simulink model "pwr_measure_testbench"  (R2012b)
settings: Solver=ode45  StartTime=0.0  StopTime=100000  RelTol=1e-3
undefined symbols (not defined in the file): ln
libraries: xbsIndex_r4 x64, simulink x1
settings Model: Creator=rng  LastModifiedBy=rng

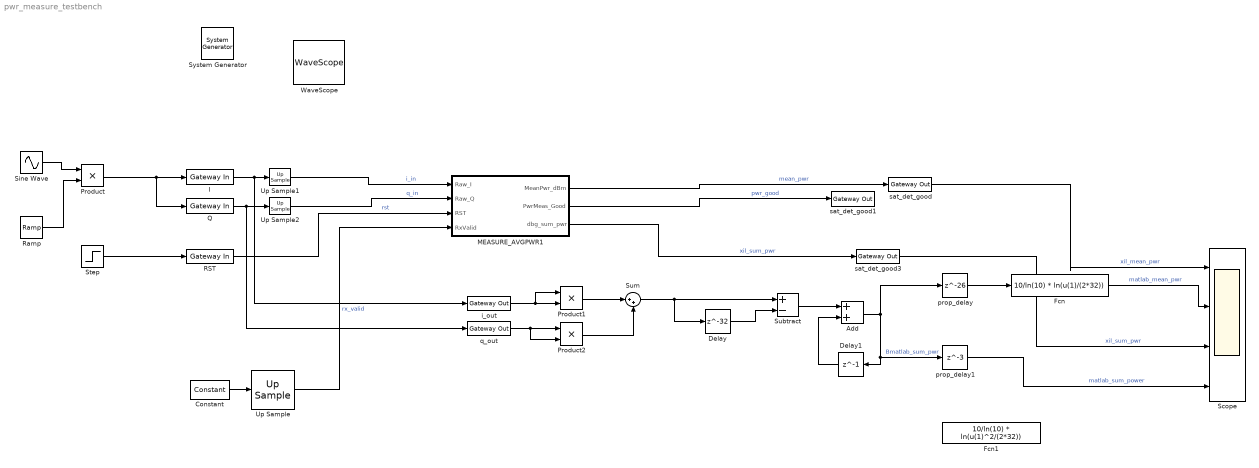
== system pwr_measure_testbench ==
  " System Generator" : xbsIndex_r4/ System Generator  Tag=genX  xilinxfamily=virtex6  part=xc6vlx240t  speed=-2  package=ff1156  synthesis_tool=XST  clock_wrapper=Clock Enables  directory=./volo_agcdc_generated_pcores  proj_type=Project Navigator  Synth_file=XST Defaults  Impl_file=ISE Defaults  testbench=off  simulink_period=1  sysclk_period=10  dcm_input_clock_period=100  incr_netlist=off  trim_vbits=Everywhere in SubSystem  dbl_ovrd=According to Block Masks  core_generation=According to Block Masks  run_coregen=off  deprecated_control=off  eval_field=0  block_type=sysgen
      settings: block_version=10.1.3
  Add : Sum
  Constant : xbsIndex_r4/Constant  const=1  gui_display_data_type=Boolean  arith_type=Boolean  n_bits=16  bin_pt=14  preci_type=Single  exp_width=8  frac_width=24  explicit_period=on  period=4  equ=P=C  opselect=C  inp2=PCIN>>17  opr=+  inp1=P  carry=CIN  dbl_ovrd=off  block_type=constant
  Delay : Delay  DelayLength=32  InitialCondition=0
  Delay1 : Delay  DelayLength=1  InitialCondition=0
  Fcn : Fcn  Expr=10/ln(10) * ln(u(1)/(2*32))
  Fcn1 : Fcn  Expr=10/ln(10) * ln(u(1)^2/(2*32))
  I : xbsIndex_r4/Gateway In  gui_display_data_type=Fixed-point  arith_type="Signed  (2's comp)"  n_bits=12  bin_pt=11  preci_type=Single  exp_width=8  frac_width=24  quantization="Round  (unbiased: +/- Inf)"  overflow=Saturate  period=4  dbl_ovrd=off  timing_constraint=None  locs_specified=off  LOCs={}  UseAsADC=off  ADCChannel='1'  inherit_from_input=off  hdl_port=on  block_type=gatewayin
  MEASURE_AVGPWR1 : Subsystem
  Product : Product  RndMeth=Zero
  Product1 : Product  RndMeth=Zero
  Product2 : Product  RndMeth=Zero
  Q : xbsIndex_r4/Gateway In  gui_display_data_type=Fixed-point  arith_type="Signed  (2's comp)"  n_bits=12  bin_pt=11  preci_type=Single  exp_width=8  frac_width=24  quantization="Round  (unbiased: +/- Inf)"  overflow=Saturate  period=4  dbl_ovrd=off  timing_constraint=None  locs_specified=off  LOCs={}  UseAsADC=off  ADCChannel='1'  inherit_from_input=off  hdl_port=on  block_type=gatewayin
  RST : xbsIndex_r4/Gateway In  gui_display_data_type=Boolean  arith_type=Boolean  n_bits=12  bin_pt=11  preci_type=Single  exp_width=8  frac_width=24  quantization="Round  (unbiased: +/- Inf)"  overflow=Saturate  period=1  dbl_ovrd=off  timing_constraint=None  locs_specified=off  LOCs={}  UseAsADC=off  ADCChannel='1'  inherit_from_input=off  hdl_port=on  block_type=gatewayin
  Ramp : simulink/Sources/Ramp  slope=0.1  start=0  X0=0
  Scope : Scope  NumInputPorts=4
      settings: YMin=0~-5~-5~-5  YMax=0.003~5~5~5
  Sine Wave : Sin  Amplitude=0.000001  Frequency=10  SampleTime=1
  Step : Step  Time=5  Before=1  After=0  SampleTime=0
  Subtract : Sum  Inputs=+-
  Sum : Sum  Inputs=|++
  Up Sample : xbsIndex_r4/Up Sample  sample_ratio=4  copy_samples=off  en=off  latency=0  dbl_ovrd=off  block_type=usamp
  Up Sample1 : xbsIndex_r4/Up Sample  sample_ratio=4  copy_samples=on  en=off  latency=0  dbl_ovrd=off  block_type=usamp
  Up Sample2 : xbsIndex_r4/Up Sample  sample_ratio=4  copy_samples=on  en=off  latency=0  dbl_ovrd=off  block_type=usamp
  WaveScope : xbsIndex_r4/WaveScope  block_type=wavescope
  i_out : xbsIndex_r4/Gateway Out  inherit_from_input=off  hdl_port=off  timing_constraint=None  locs_specified=off  LOCs={}  UseAsDAC=off  DACChannel='1'  block_type=gatewayout
  prop_delay : Delay  DelayLength=26  InitialCondition=0
  prop_delay1 : Delay  DelayLength=3  InitialCondition=0
  q_out : xbsIndex_r4/Gateway Out  inherit_from_input=off  hdl_port=off  timing_constraint=None  locs_specified=off  LOCs={}  UseAsDAC=off  DACChannel='1'  block_type=gatewayout
  sat_det_good : xbsIndex_r4/Gateway Out  inherit_from_input=off  hdl_port=off  timing_constraint=None  locs_specified=off  LOCs={}  UseAsDAC=off  DACChannel='1'  block_type=gatewayout
  sat_det_good1 : xbsIndex_r4/Gateway Out  inherit_from_input=off  hdl_port=off  timing_constraint=None  locs_specified=off  LOCs={}  UseAsDAC=off  DACChannel='1'  block_type=gatewayout
  sat_det_good3 : xbsIndex_r4/Gateway Out  inherit_from_input=off  hdl_port=off  timing_constraint=None  locs_specified=off  LOCs={}  UseAsDAC=off  DACChannel='1'  block_type=gatewayout
  wires:
  I/1 -> i_out/1, Up Sample1/1
  Q/1 -> q_out/1, Up Sample2/1
  Constant/1 -> Up Sample/1
  Up Sample/1 -> MEASURE_AVGPWR1/4(RxValid)  "rx_valid"
  Up Sample1/1 -> MEASURE_AVGPWR1/1(Raw_I)  "i_in"
  Up Sample2/1 -> MEASURE_AVGPWR1/2(Raw_Q)  "q_in"
  Product/1 -> Q/1, I/1
  Sine Wave/1 -> Product/1
  Ramp/1 -> Product/2
  Step/1 -> RST/1
  MEASURE_AVGPWR1/1(MeanPwr_dBm) -> sat_det_good/1  "mean_pwr"
  MEASURE_AVGPWR1/2(PwrMeas_Good) -> sat_det_good1/1  "pwr_good"
  RST/1 -> MEASURE_AVGPWR1/3(RST)  "rst"
  i_out/1 -> Product1/2, Product1/1
  q_out/1 -> Product2/2, Product2/1
  Product1/1 -> Sum/1
  Product2/1 -> Sum/2
  Delay/1 -> Subtract/2
  Sum/1 -> Subtract/1, Delay/1
  Subtract/1 -> Add/1
  Add/1 -> Delay1/1, prop_delay1/1, prop_delay/1  "Bmatlab_sum_pwr"
  Delay1/1 -> Add/2
  Fcn/1 -> Scope/2  "matlab_mean_pwr"
  sat_det_good/1 -> Scope/1  "xil_mean_pwr"
  MEASURE_AVGPWR1/3(dbg_sum_pwr) -> sat_det_good3/1  "xil_sum_pwr"
  prop_delay/1 -> Fcn/1
  prop_delay1/1 -> Scope/4  "matlab_sum_power"
  sat_det_good3/1 -> Scope/3  "xil_sum_pwr"

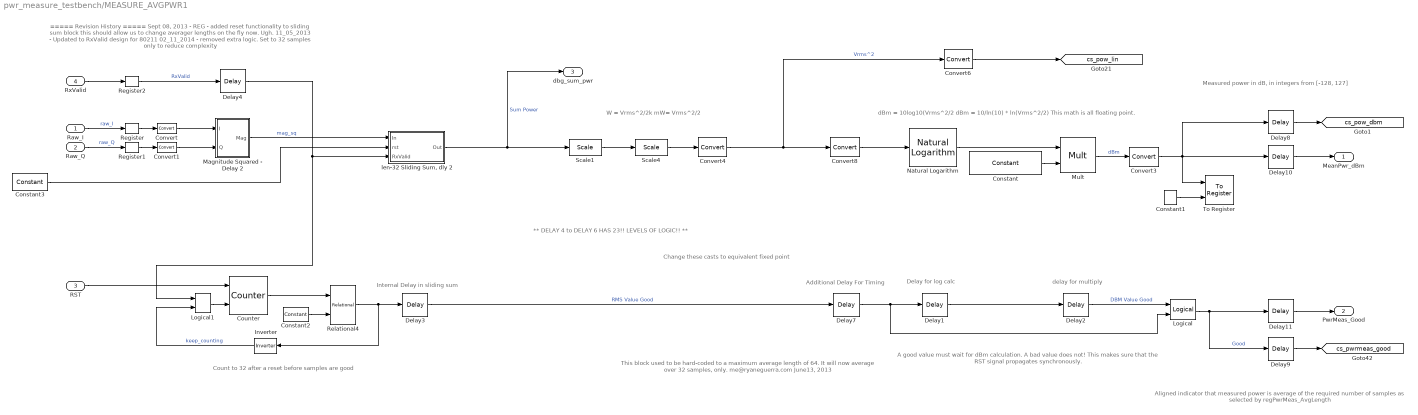
== system pwr_measure_testbench/MEASURE_AVGPWR1 ==
  note: delay for multiply
  note: Delay for log calc
  note: Count to 32 after a reset before samples are good
  note: Change these casts to equivalent fixed point
  note: ** DELAY 4 to DELAY 6 HAS 23!! LEVELS OF LOGIC!! **
  note: Additional Delay For Timing
  note: Internal Delay in sliding sum
  note: ===== Revision History =====
      | Sept 08, 2013 - REG - added reset functionality to sliding sum block
      | this should allow us to change averager lengths on the fly now. Ugh.
      | 11_05_2013 - Updated to RxValid design for 80211
      | 02_11_2014 - removed extra logic. Set to 32 samples only to reduce complexity
  note: A good value must wait for dBm calculation.
      | A bad value does not! This makes sure that
      | the RST signal propagates synchronously.
  note: Aligned indicator that
      | measured power is average
      | of the required number
      | of samples as selected
      | by regPwrMeas_AvgLength
  note: Measured power in dB,
      | in  integers from
      | [-128, 127]
  note: dBm = 10log10(Vrms^2/2
      | dBm = 10/ln(10) * ln(Vrms^2/2)
      | This math is all floating point.
  note: W = Vrms^2/2k
      | mW= Vrms^2/2
  note: This block used to be hard-coded to a maximum average length of 64.
      | It will now average over 32 samples, only.
      | me@ryaneguerra.com
      | June13, 2013
  Raw_I : Inport
  Raw_Q : Inport  Port=2
  RST : Inport  Port=3
  RxValid : Inport  Port=4
  Constant : xbsIndex_r4/Constant  const=10/log(10)  gui_display_data_type=Floating-point  arith_type=Floating-point  n_bits=18  bin_pt=14  preci_type=Single  exp_width=8  frac_width=24  explicit_period=on  period=1  equ=P=C  opselect=C  inp2=PCIN>>17  opr=+  inp1=P  carry=CIN  dbl_ovrd=off  block_type=constant
  Constant1 : xbsIndex_r4/Constant  const=1  gui_display_data_type=Boolean  arith_type=Boolean  n_bits=18  bin_pt=14  preci_type=Single  exp_width=8  frac_width=24  explicit_period=on  period=1  equ=P=C  opselect=C  inp2=PCIN>>17  opr=+  inp1=P  carry=CIN  dbl_ovrd=off  block_type=constant
  Constant2 : xbsIndex_r4/Constant  const=32  gui_display_data_type=Fixed-point  arith_type=Unsigned  n_bits=6  bin_pt=0  preci_type=Single  exp_width=8  frac_width=24  explicit_period=on  period=1  equ=P=C  opselect=C  inp2=PCIN>>17  opr=+  inp1=P  carry=CIN  dbl_ovrd=off  block_type=constant
  Constant3 : xbsIndex_r4/Constant  const=0  gui_display_data_type=Boolean  arith_type=Boolean  n_bits=16  bin_pt=14  preci_type=Single  exp_width=8  frac_width=24  explicit_period=on  period=1  equ=P=C  opselect=C  inp2=PCIN>>17  opr=+  inp1=P  carry=CIN  dbl_ovrd=off  block_type=constant
  Convert : xbsIndex_r4/Convert  gui_display_data_type=Fixed-point  arith_type="Signed  (2's comp)"  n_bits=12  bin_pt=11  float_type=Single  exp_bits=8  fraction_bits=24  quantization=Truncate  overflow=Wrap  en=off  latency=0  dbl_ovrd=off  pipeline=off  block_type=convert
  Convert1 : xbsIndex_r4/Convert  gui_display_data_type=Fixed-point  arith_type="Signed  (2's comp)"  n_bits=12  bin_pt=11  float_type=Single  exp_bits=8  fraction_bits=24  quantization=Truncate  overflow=Wrap  en=off  latency=0  dbl_ovrd=off  pipeline=off  block_type=convert
  Convert3 : xbsIndex_r4/Convert  gui_display_data_type=Fixed-point  arith_type="Signed  (2's comp)"  n_bits=9  bin_pt=0  float_type=Single  exp_bits=8  fraction_bits=24  quantization="Round  (unbiased: +/- Inf)"  overflow=Saturate  en=off  latency=0  dbl_ovrd=off  pipeline=off  block_type=convert
  Convert4 : xbsIndex_r4/Convert  gui_display_data_type=Fixed-point  arith_type="Signed  (2's comp)"  n_bits=34  bin_pt=22  float_type=Single  exp_bits=8  fraction_bits=24  quantization=Truncate  overflow=Wrap  en=off  latency=0  dbl_ovrd=off  pipeline=off  block_type=convert
  Convert6 : xbsIndex_r4/Convert  gui_display_data_type=Fixed-point  arith_type="Signed  (2's comp)"  n_bits=32  bin_pt=15  float_type=Single  exp_bits=8  fraction_bits=24  quantization="Round  (unbiased: +/- Inf)"  overflow=Saturate  en=off  latency=0  dbl_ovrd=off  pipeline=off  block_type=convert
  Convert8 : xbsIndex_r4/Convert  gui_display_data_type=Floating-point  arith_type=Floating-point  n_bits=34  bin_pt=22  float_type=Single  exp_bits=8  fraction_bits=24  quantization=Truncate  overflow=Wrap  en=off  latency=3  dbl_ovrd=off  pipeline=on  block_type=convert
  Counter : xbsIndex_r4/Counter  cnt_type=Free Running  cnt_to=10  operation=Up  start_count=0  cnt_by_val=1  arith_type=Unsigned  n_bits=10  bin_pt=0  load_pin=off  rst=on  en=on  explicit_period=on  period=1  dbl_ovrd=off  use_behavioral_HDL=off  implementation=Fabric  block_type=counter
  Delay1 : xbsIndex_r4/Delay  rst=off  infoeditControl=Selection of Reset will increase slice count due to use of real FFs and instead of SRLs  en=off  latency=6  dbl_ovrd=off  reg_retiming=off  block_type=delay
  Delay{8..11} (4 alike) : xbsIndex_r4/Delay  rst=off  infoeditControl=Selection of Reset will increase slice count due to use of real FFs and instead of SRLs  en=off  latency=1  dbl_ovrd=off  reg_retiming=off  block_type=delay
  Delay2 : xbsIndex_r4/Delay  rst=off  infoeditControl=Selection of Reset will increase slice count due to use of real FFs and instead of SRLs  en=off  latency=6  dbl_ovrd=off  reg_retiming=off  block_type=delay
  Delay3 : xbsIndex_r4/Delay  rst=off  infoeditControl=Selection of Reset will increase slice count due to use of real FFs and instead of SRLs  en=off  latency=2  dbl_ovrd=off  reg_retiming=off  block_type=delay
  Delay4 : xbsIndex_r4/Delay  rst=off  infoeditControl=Selection of Reset will increase slice count due to use of real FFs and instead of SRLs  en=off  latency=2  dbl_ovrd=off  reg_retiming=off  block_type=delay
  Delay7 : xbsIndex_r4/Delay  rst=off  infoeditControl=Selection of Reset will increase slice count due to use of real FFs and instead of SRLs  en=off  latency=3  dbl_ovrd=off  reg_retiming=off  block_type=delay
  Inverter : xbsIndex_r4/Inverter  en=off  latency=0  dbl_ovrd=off  block_type=inv
  Logical : xbsIndex_r4/Logical  logical_function=AND  inputs=2  en=off  latency=0  precision=Full  arith_type=Unsigned  n_bits=16  bin_pt=0  align_bp=on  dbl_ovrd=off  block_type=logical
  Logical1 : xbsIndex_r4/Logical  logical_function=AND  inputs=2  en=off  latency=0  precision=Full  arith_type=Unsigned  n_bits=16  bin_pt=0  align_bp=on  dbl_ovrd=off  block_type=logical
  Magnitude Squared - Delay 2 : Subsystem
  Mult : xbsIndex_r4/Mult  precision=Full  arith_type="Signed  (2's comp)"  n_bits=8  bin_pt=0  quantization=Truncate  overflow=Saturate  en=off  latency=6  dbl_ovrd=off  use_behavioral_HDL=off  opt=Speed  use_embedded=on  optimum_pipeline=off  pipeline=on  use_rpm=on  placement_style=Triangular  block_type=mult
  Natural Logarithm : xbsIndex_r4/Natural Logarithm  flow_control=NonBlocking  axi_optimize_goal=Resources  latency=6  has_a_tlast=off  has_a_tuser=off  en=off  has_result_tready=off  has_invalid_op=off  has_divide_by_zero=off  fpo_op_type=log_base_e  rate=1  has_b_tlast=false  has_b_tuser=false  result_tlast_behv=1  has_underflow=false  has_overflow=false  block_type=natlog
      settings: infoedit=Blocking: Wait for data on all inputs, allow back-pressure.<br>NonBlocking: operate every cycle in which all inputs are valid, no back-pressure.
  Register : xbsIndex_r4/Register  init=0  rst=off  en=off  dbl_ovrd=off  block_type=register
  Register1 : xbsIndex_r4/Register  init=0  rst=off  en=off  dbl_ovrd=off  block_type=register
  Register2 : xbsIndex_r4/Register  init=0  rst=off  en=off  dbl_ovrd=off  block_type=register
  Relational4 : xbsIndex_r4/Relational  mode=a=b  en=off  latency=0  dbl_ovrd=off  block_type=relational
  Scale1 : xbsIndex_r4/Scale  scale_factor=-5  dbl_ovrd=off  block_type=scale
  Scale4 : xbsIndex_r4/Scale  scale_factor=-1  dbl_ovrd=off  block_type=scale
  To Register : xbsIndex_r4/To Register  shared_memory_name='regWSD_meanPower'  init=0  ownership=Locally owned and initialized  explicit_data_type=on  gui_display_data_type=Fixed-point  arith_type="Signed  (2's comp)"  n_bits=9  bin_pt=0  preci_type=Single  dbl_ovrd=off  block_type=toreg
      settings: AttributesFormatString=<< %<shared_memory_name> >>  infoedit="Register block that writes data to a shared memory register.  Delay of one sample period."
  "len-32 Sliding Sum, dly 2" : Subsystem
  MeanPwr_dBm : Outport
  PwrMeas_Good : Outport  Port=2
  dbg_sum_pwr : Outport  Port=3
  tag scope: cs_pow_dbm=global, cs_pow_lin=global, cs_pwrmeas_good=global
  wires:
  Magnitude Squared - Delay 2/1(Mag) -> "len-32 Sliding Sum, dly 2"/1(In)  "mag_sq"
  "len-32 Sliding Sum, dly 2"/1(Out) -> dbg_sum_pwr/1, Scale1/1  "Sum Power"
  Raw_I/1 -> Register/1  "raw_I"
  Raw_Q/1 -> Register1/1  "raw_Q"
  Relational4/1 -> Delay3/1, Inverter/1
  Counter/1 -> Relational4/1
  Inverter/1 -> Logical1/2  "keep_counting"
  Convert/1 -> Magnitude Squared - Delay 2/1(I)
  Convert1/1 -> Magnitude Squared - Delay 2/2(Q)
  Convert4/1 -> Convert8/1, Convert6/1  "Vrms^2"
  Natural Logarithm/1 -> Mult/1
  Constant/1 -> Mult/2
  Mult/1 -> Convert3/1  "dBm"
  Convert3/1 -> Delay10/1, Delay8/1, To Register/1
  Delay2/1 -> Logical/1  "DBM Value Good"
  Logical/1 -> Delay11/1, Delay9/1  "Good"
  Scale1/1 -> Scale4/1
  Scale4/1 -> Convert4/1
  Convert6/1 -> [cs_pow_lin]
  Constant3/1 -> "len-32 Sliding Sum, dly 2"/2(rst)
  Constant1/1 -> To Register/2
  Register/1 -> Convert/1
  Register1/1 -> Convert1/1
  RST/1 -> Counter/1
  RxValid/1 -> Register2/1
  Register2/1 -> Delay4/1  "RxValid"
  Logical1/1 -> Counter/2
  Delay1/1 -> Delay2/1
  Delay3/1 -> Delay7/1  "RMS Value Good"
  Convert8/1 -> Natural Logarithm/1
  Delay7/1 -> Logical/2, Delay1/1
  Delay8/1 -> [cs_pow_dbm]
  Delay9/1 -> [cs_pwrmeas_good]
  Delay10/1 -> MeanPwr_dBm/1
  Delay11/1 -> PwrMeas_Good/1
  Constant2/1 -> Relational4/2
  Delay4/1 -> Logical1/1, "len-32 Sliding Sum, dly 2"/3(RxValid)

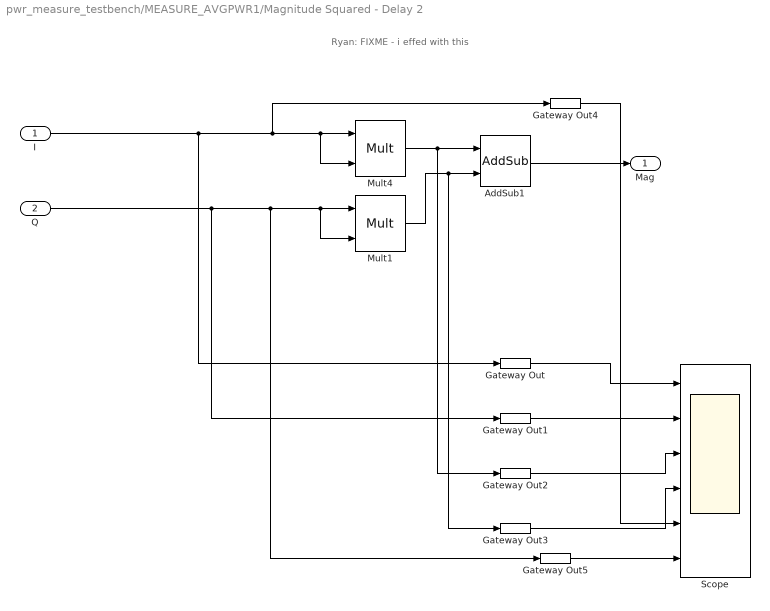
== system pwr_measure_testbench/MEASURE_AVGPWR1/Magnitude Squared - Delay 2 ==
  note: Ryan: FIXME - i effed with this
  I : Inport
  Q : Inport  Port=2
  AddSub1 : xbsIndex_r4/AddSub  mode=Addition  use_carryin=off  use_carryout=off  en=off  latency=1  precision=Full  arith_type=Unsigned  n_bits=16  bin_pt=15  quantization=Truncate  overflow=Saturate  dbl_ovrd=off  use_behavioral_HDL=on  hw_selection=Fabric  pipelined=off  use_rpm=on  block_type=addsub
      settings: xl_area=[12 22 0 22 0 0 0]  block_version=VER_STRING_GOES_HERE
  Gateway Out{,1..5} (6 alike) : xbsIndex_r4/Gateway Out  inherit_from_input=off  hdl_port=off  timing_constraint=None  locs_specified=off  LOCs={}  UseAsDAC=off  DACChannel='1'  block_type=gatewayout
  Mult1 : xbsIndex_r4/Mult  precision=Full  arith_type=Unsigned  n_bits=16  bin_pt=16  quantization=Truncate  overflow=Saturate  en=off  latency=1  dbl_ovrd=off  use_behavioral_HDL=off  opt=Speed  use_embedded=on  optimum_pipeline=off  pipeline=on  use_rpm=off  placement_style=Rectangular shape  block_type=mult
      settings: xl_area=[63 105 0 106 0 4 0]  block_version=VER_STRING_GOES_HERE
  Mult4 : xbsIndex_r4/Mult  precision=Full  arith_type=Unsigned  n_bits=16  bin_pt=16  quantization=Truncate  overflow=Saturate  en=off  latency=1  dbl_ovrd=off  use_behavioral_HDL=off  opt=Speed  use_embedded=on  optimum_pipeline=off  pipeline=on  use_rpm=off  placement_style=Rectangular shape  block_type=mult
      settings: xl_area=[63 105 0 106 0 4 0]  block_version=VER_STRING_GOES_HERE
  Scope : Scope  NumInputPorts=6
      settings: ShowLegends=on  YMin=-5~-5~-5~-5~-5~-5  YMax=5~5~5~5~5~5  SaveName=ScopeData5
  Mag : Outport
  wires:
  AddSub1/1 -> Mag/1
  Mult1/1 -> Gateway Out3/1, AddSub1/2
  Mult4/1 -> Gateway Out2/1, AddSub1/1
  Gateway Out/1 -> Scope/1
  Gateway Out1/1 -> Scope/2
  Gateway Out2/1 -> Scope/3
  Gateway Out3/1 -> Scope/4
  I/1 -> Gateway Out4/1, Mult4/2, Mult4/1, Gateway Out/1
  Q/1 -> Gateway Out5/1, Mult1/1, Mult1/2, Gateway Out1/1
  Gateway Out4/1 -> Scope/5
  Gateway Out5/1 -> Scope/6

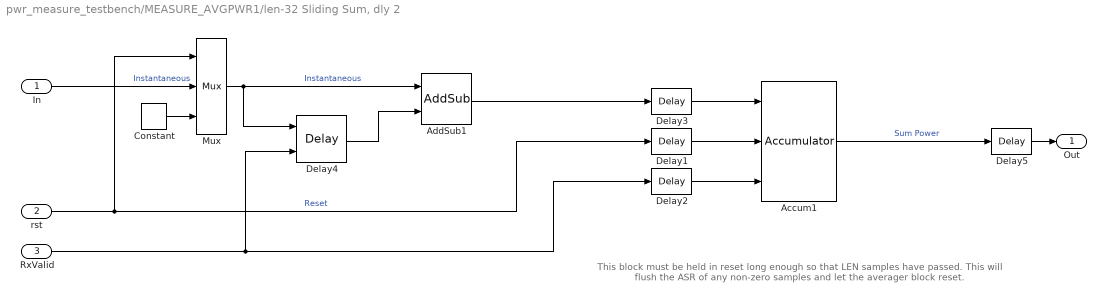
== system pwr_measure_testbench/MEASURE_AVGPWR1/len-32 Sliding Sum, dly 2 ==
  note: This block must be held in reset long enough so that LEN samples have passed.
      | This will flush the ASR of any non-zero samples and let the averager block reset.
  In : Inport
  rst : Inport  Port=2
  RxValid : Inport  Port=3
  Accum1 : xbsIndex_r4/Accumulator  operation=Add  n_bits=32  overflow=Saturate  scale=1  rst=on  infoeditControl=reset for floating point data type must be asserted for a minimum of 2 cycles  hasbypass=off  en=on  latency=0  dbl_ovrd=off  msb_inp=100  msb=100  lsb=-100  use_behavioral_HDL=on  implementation=Fabric  block_type=accum
      settings: xl_area=[12 23 0 22 0 0 0]  block_version=VER_STRING_GOES_HERE
  AddSub1 : xbsIndex_r4/AddSub  mode=Subtraction  use_carryin=off  use_carryout=off  en=off  latency=0  precision=Full  arith_type="Signed  (2's comp)"  n_bits=36  bin_pt=28  quantization=Truncate  overflow=Saturate  dbl_ovrd=off  use_behavioral_HDL=on  hw_selection=Fabric  pipelined=off  use_rpm=off  block_type=addsub
      settings: xl_area=[9 18 0 17 0 0 0]  block_version=VER_STRING_GOES_HERE
  Constant : xbsIndex_r4/Constant  const=0  gui_display_data_type=Fixed-point  arith_type=Signed (2's comp)  n_bits=16  bin_pt=14  preci_type=Single  exp_width=8  frac_width=24  explicit_period=off  period=1  equ=P=C  opselect=C  inp2=PCIN>>17  opr=+  inp1=P  carry=CIN  dbl_ovrd=off  block_type=constant
  Delay{1..3,5} (4 alike) : xbsIndex_r4/Delay  rst=off  infoeditControl=Selection of Reset will increase slice count due to use of real FFs and instead of SRLs  en=off  latency=1  dbl_ovrd=off  reg_retiming=off  block_type=delay
  Delay4 : xbsIndex_r4/Delay  rst=off  infoeditControl=Selection of Reset will increase slice count due to use of real FFs and instead of SRLs  en=on  latency=32  dbl_ovrd=off  reg_retiming=off  block_type=delay
  Mux : xbsIndex_r4/Mux  inputs=2  en=off  latency=0  precision=Full  arith_type=Unsigned  n_bits=16  bin_pt=14  quantization=Truncate  overflow=Wrap  dbl_ovrd=off  block_type=mux
  Out : Outport
  wires:
  Delay4/1 -> AddSub1/2
  AddSub1/1 -> Delay3/1
  Mux/1 -> Delay4/1, AddSub1/1  "Instantaneous"
  Accum1/1 -> Delay5/1  "Sum Power"
  rst/1 -> Mux/1, Delay1/1  "Reset"
  In/1 -> Mux/2  "Instantaneous"
  Constant/1 -> Mux/3
  RxValid/1 -> Delay4/2, Delay2/1
  Delay3/1 -> Accum1/1
  Delay1/1 -> Accum1/2
  Delay2/1 -> Accum1/3
  Delay5/1 -> Out/1
